simulink model "func1_b"  (R2023a)
settings: Solver=VariableStepAuto  StartTime=0.0  StopTime=10.0  RelTol=1e-3  EnableMultiTasking=on
libraries: vmcUtilities x2, hlsBasic x1, parametrization_1_lib x1
settings Model: Creator=abehbood  LastModifiedBy=robg
settings SolverCC: AlgebraicLoopSolver=TrustRegion
settings DataIOCC: ReturnWorkspaceOutputs=off
settings OptimizationCC: LifeSpan=inf
settings DebuggingCC: UnconnectedInputMsg=warning  UnconnectedOutputMsg=warning  UnconnectedLineMsg=warning  SFUnexpectedBacktrackingDiag=warning  SFNoUnconditionalDefaultTransitionDiag=warning  ArithmeticOperatorsInVariantConditions=warning
settings ModelReferenceCC: EnableRefExpFcnMdlSchedulingChecks=on
settings SFSimCC: SimUseLocalCustomCode=off  CustomCodeUndefinedFunction=UseInterfaceOnly
settings RTWCC: RTWUseLocalCustomCode=off  DLArmComputeVersion=19.05
settings CodeAppCC: StateflowObjectComments=on
settings GRTTargetCC: TargetLangStandard=C89/C90 (ANSI)
settings ConfigComp: CovMetricSettings=dw  CovSaveCumulativeToWorkspaceVar=on  CovSaveSingleToWorkspaceVar=on  CovExternalEMLEnable=off

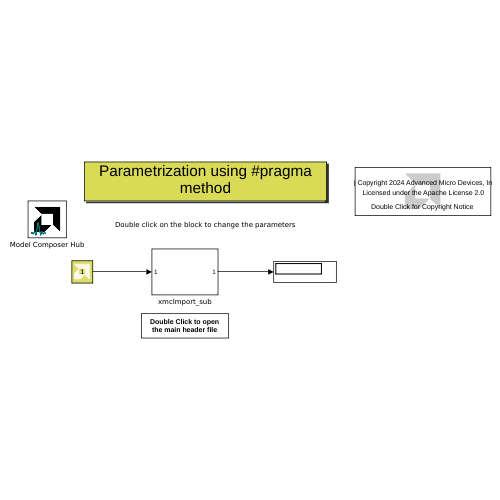
[thumbnail: Simulink's stored preview of the top-level diagram]
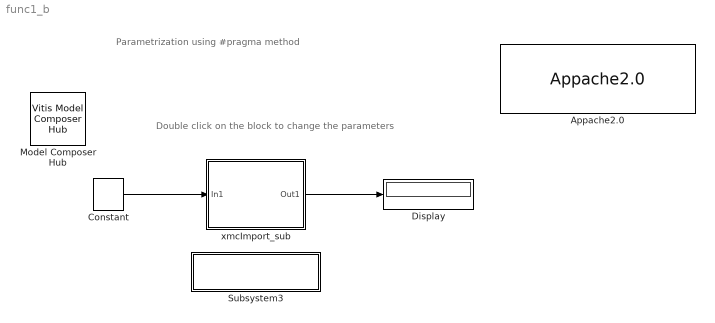
== system func1_b ==
  note: Double click on the block to change the parameters
  note: Parametrization using #pragma method
  Appache2.0 : vmcUtilities/Appache2.0
  Constant : hlsBasic/Constant  Value=1  VectorParams1D=off  SampleTime=1.0  OutDataType=int16  TypeExp=''  Signedness=Signed  WordLength=16  FractionalLength=0  RoundingMode=Truncation to minus infinity  OverflowMode=Wrap around
  Display : Display
  Model Composer Hub : vmcUtilities/Vitis Model Composer Hub  Tag=genX  CodeGeneration=off  SubsystemName=xmcImport_sub  StartColumn=1  NumberOfColumns=1  TargetDirectory=./code  exportDesign=off  analyzeDesign=off  validateDesignOnHw=off  ExportType=IP Catalog  IpVendor=xilinx.com  IpLibrary=hls  IpVersion=1.0  IpHWLanguage=Verilog  AieCompilerOptions={}  AieSimulatorOptions={}  CreateTestbench=off  TestbenchStackSize=10  RunRtlSim=off  RunCSim=off  RunAieSim=off  AieSimTimeout=50000  RunAieSimProfiling=off  LaunchVitisAnalyzer=off  PlotOutput=off  RunX86Sim=off  X86SimTimeout=10  GenHwImage=off  GenLibadfXo=off  GenHwValidationCode=off  PlatformType=Not Specified  HwSystemType=Baremetal  HwValidationTarget=hw  ProjDevice=xcku11p-ffva1156-1-e  ProjDevicePart=xcku11p-ffva1156-1-e  SamplePeriod=-1  ClockFrequency=200  DataPathParallelism=1  xilinxfamily=Kintex7  part=xc7k325t  speed=-3  package=fbg676  directory=./netlist  testbench=off  incr_netlist=off  synthesis_tool=Vivado  clock_wrapper=Clock Enables  dbl_ovrd=According to Block Masks  dcm_input_clock_period=10  sysclk_period=10  simulink_period=1  eval_field=0  LogFileName=''  NThreads=4
  Subsystem3 : Subsystem
      settings: OpenFcn=xmcOpenFileEx
      mask Display: disp(sprintf('Double Click to open\nthe main header file'))
  xmcImport_sub : Subsystem
  wires:
  Constant/1 -> xmcImport_sub/1(In1)
  xmcImport_sub/1(Out1) -> Display/1

== system func1_b/Subsystem3 ==

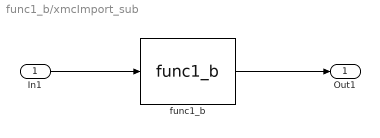
== system func1_b/xmcImport_sub ==
  In1 : Inport
  func1_b : parametrization_1_lib/func1_b  LibraryFunction=func1_b  IncludeFiles={'func1_b.h'}  SourceFiles={}  IncludeDirectories={}  TemplateParams={' '}  FunctionParamTypes={xmcDataType('void'); xmcDataType('int16_t'); xmcDataType('int8_t &'); xmcDataType('double'); xmcDataType('int8_t')}  FunctionParamPassbys={0.000000000000000000e+00; 0.000000000000000000e+00; 1.000000000000000000e+00; 0.000000000000000000e+00; 0.000000000000000000e+00}  FunctionParamDimensions={'1'; '1'; '1'; '1'; '1'}  FunctionParamNames={'return'; 'in'; 'out'; 'P1'; 'P2'}  FunctionParamDir={0.000000000000000000e+00; 1.000000000000000000e+00; 2.000000000000000000e+00; 3.000000000000000000e+00; 3.000000000000000000e+00}  FunctionParamSupportsStreaming={false; false; false; false; false}  BufferDepth={'0'}  FunctionParamValues={'0'; '0'; '0'; '0'; '10'}  ThroughputFactors={''}  P1=0  P2=10
  Out1 : Outport
  wires:
  func1_b/1 -> Out1/1
  In1/1 -> func1_b/1
